simulink model "lab7_t15"  (R2021a)
settings: Solver=VariableStepAuto  StartTime=0.0  StopTime=10.0  RelTol=1e-3
settings Model: Creator=reemb  LastModifiedBy=reemb

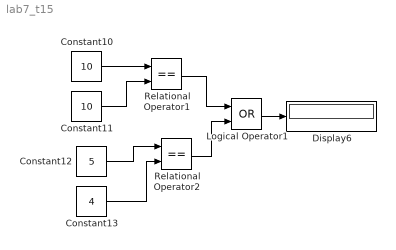
== system lab7_t15 ==
  Constant10 : Constant  Value=10
  Constant11 : Constant  Value=10
  Constant12 : Constant  Value=5
  Constant13 : Constant  Value=4
  Display6 : Display
  Logical Operator1 : Logic  Operator=OR  AllPortsSameDT=off  OutDataTypeStr=boolean
  Relational Operator1 : RelationalOperator  Operator===  OutDataTypeStr=boolean  RndMeth=Simplest
  Relational Operator2 : RelationalOperator  Operator===  OutDataTypeStr=boolean  RndMeth=Simplest
  wires:
  Constant10/1 -> Relational Operator1/1
  Constant13/1 -> Relational Operator2/2
  Constant12/1 -> Relational Operator2/1
  Relational Operator2/1 -> Logical Operator1/2
  Relational Operator1/1 -> Logical Operator1/1
  Logical Operator1/1 -> Display6/1
  Constant11/1 -> Relational Operator1/2
